simulink model "IMC_Ex1_simulink"  (R2018b)
settings: Solver=VariableStepAuto  StartTime=0.0  StopTime=4  RelTol=1e-3
values from neighbouring files (symbols this model uses):
  Kc = vars(5)    [Optimum.m]
  N = vars(4)    [CC.m]    (also in CHR.m; Optimum.m; PID_1.m = 10; PID_10.m = 10)
  Td = ((0.27-0.36*tau)/(1-0.87*tau)) * L    [CC.m]    (also in CHR.m = KK(typ, 6) * L; FOIPDT.m = T; IPDT.m = a(iC, 5) * L; Optimum.m = 0.144 * Tc)
  Ti = ((2.5-2*tau)/(1-0.39*tau)) * L    [CC.m]    (also in CHR.m = KK(typ, 5) * TT; FOIPDT.m = 2 * L * (1+a); IPDT.m = a(iC, 4) * L; Optimum.m = Tc * (1.751*kappa-0.612) / (3.776*kappa+1.388))
undefined symbols (not defined in the file or in its folder): b, c, N0, Tt, Tt0
settings Model: Creator=Erfan Etesami  LastModifiedBy=Erfan Etesami

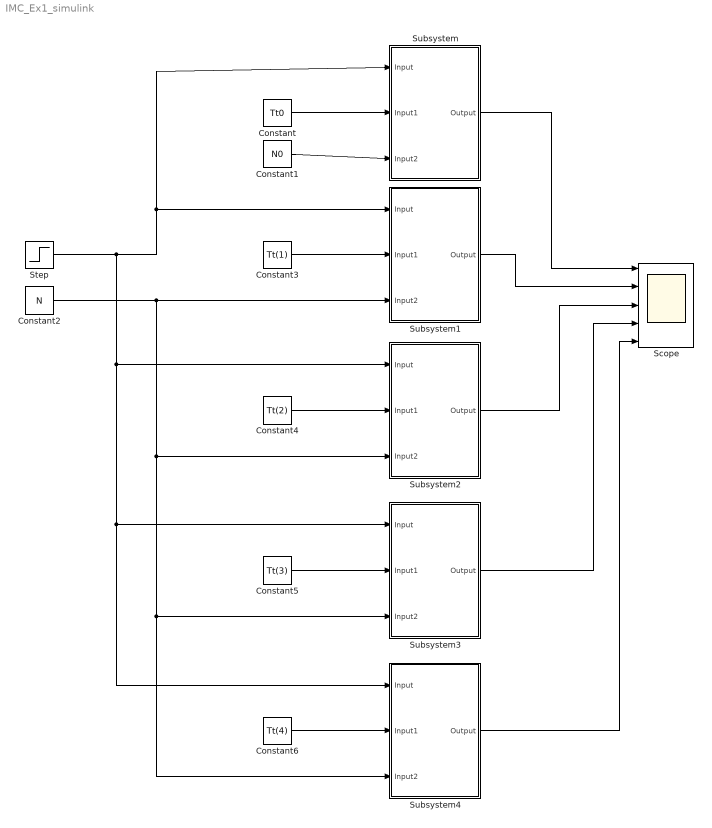
== system IMC_Ex1_simulink ==
  Constant : Constant  Value=Tt0
  Constant1 : Constant  Value=N0
  Constant2 : Constant  Value=N
  Constant3 : Constant  Value=Tt(1)
  Constant4 : Constant  Value=Tt(2)
  Constant5 : Constant  Value=Tt(3)
  Constant6 : Constant  Value=Tt(4)
  Scope : Scope  NumInputPorts=5
  Step : Step  Time=0  SampleTime=0
  Subsystem : Subsystem
  Subsystem1 : Subsystem
  Subsystem2 : Subsystem
  Subsystem3 : Subsystem
  Subsystem4 : Subsystem
  wires:
  Subsystem/1(Output) -> Scope/1
  Step/1 -> Subsystem/1(Input), Subsystem1/1(Input), Subsystem2/1(Input), Subsystem4/1(Input), Subsystem3/1(Input)
  Constant/1 -> Subsystem/2(Input1)
  Constant1/1 -> Subsystem/3(Input2)
  Constant2/1 -> Subsystem1/3(Input2), Subsystem2/3(Input2), Subsystem4/3(Input2), Subsystem3/3(Input2)
  Constant3/1 -> Subsystem1/2(Input1)
  Constant4/1 -> Subsystem2/2(Input1)
  Subsystem1/1(Output) -> Scope/2
  Subsystem2/1(Output) -> Scope/3
  Constant5/1 -> Subsystem3/2(Input1)
  Subsystem3/1(Output) -> Scope/4
  Constant6/1 -> Subsystem4/2(Input1)
  Subsystem4/1(Output) -> Scope/5

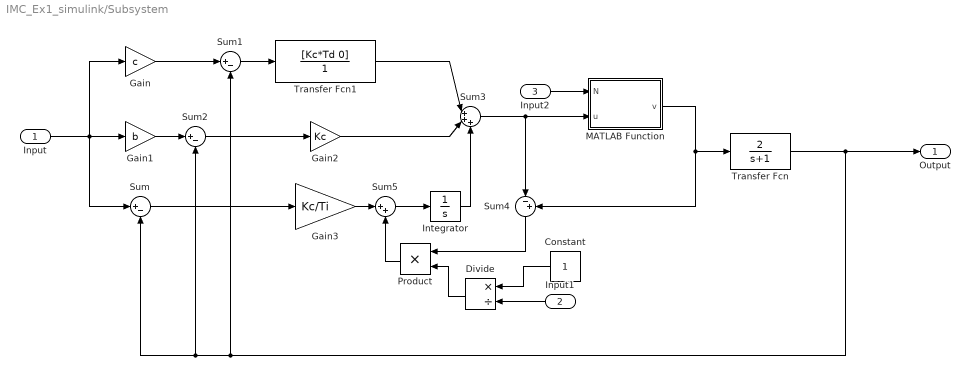
== system IMC_Ex1_simulink/Subsystem ==
  Input : Inport
  Input1 : Inport  Port=2
  Input2 : Inport  Port=3
  Constant : Constant
  Divide : Product  Inputs=*/
  Gain : Gain  Gain=c
  Gain1 : Gain  Gain=b
  Gain2 : Gain  Gain=Kc
  Gain3 : Gain  Gain=Kc/Ti
  Integrator : Integrator
  MATLAB Function : MATLAB Function  TreatAsAtomicUnit=on
  Product : Product
  Sum : Sum  Inputs=|+-
  Sum1 : Sum  Inputs=|+-
  Sum2 : Sum  Inputs=|+-
  Sum3 : Sum  Inputs=|+++
  Sum4 : Sum  Inputs=|-+
  Sum5 : Sum  Inputs=|++
  Transfer Fcn : TransferFcn  Numerator=[2]  Denominator=[1 1]
  Transfer Fcn1 : TransferFcn  Numerator=[Kc*Td 0]  Denominator=[1]
  Output : Outport
  wires:
  Product/1 -> Sum5/2
  Divide/1 -> Product/2
  Transfer Fcn/1 -> Output/1, Sum1/2, Sum2/2, Sum/2
  Input1/1 -> Divide/2
  MATLAB Function/1(v) -> Sum4/2, Transfer Fcn/1
  Input/1 -> Gain/1, Sum/1, Gain1/1
  Sum3/1 -> MATLAB Function/2(u), Sum4/1
  Transfer Fcn1/1 -> Sum3/1
  Gain/1 -> Sum1/1
  Constant/1 -> Divide/1
  Sum5/1 -> Integrator/1
  Sum4/1 -> Product/1
  Sum2/1 -> Gain2/1
  Gain3/1 -> Sum5/1
  Gain1/1 -> Sum2/1
  Integrator/1 -> Sum3/3
  Gain2/1 -> Sum3/2
  Sum/1 -> Gain3/1
  Sum1/1 -> Transfer Fcn1/1
  Input2/1 -> MATLAB Function/1(N)

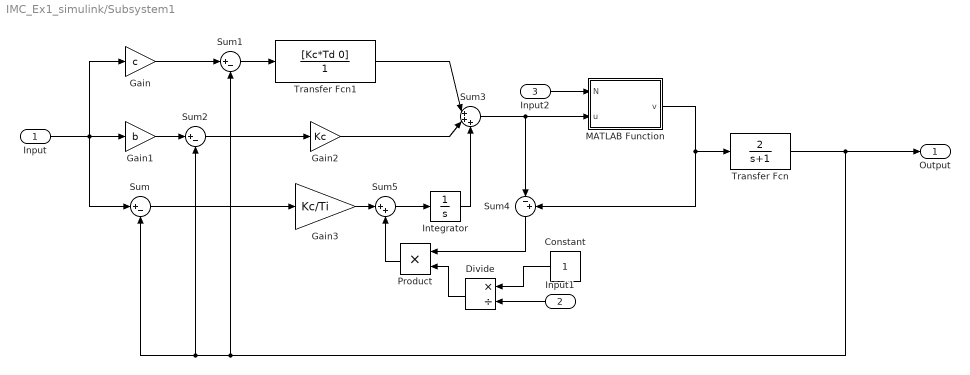
== system IMC_Ex1_simulink/Subsystem1 ==
  Input : Inport
  Input1 : Inport  Port=2
  Input2 : Inport  Port=3
  Constant : Constant
  Divide : Product  Inputs=*/
  Gain : Gain  Gain=c
  Gain1 : Gain  Gain=b
  Gain2 : Gain  Gain=Kc
  Gain3 : Gain  Gain=Kc/Ti
  Integrator : Integrator
  MATLAB Function : MATLAB Function  TreatAsAtomicUnit=on
  Product : Product
  Sum : Sum  Inputs=|+-
  Sum1 : Sum  Inputs=|+-
  Sum2 : Sum  Inputs=|+-
  Sum3 : Sum  Inputs=|+++
  Sum4 : Sum  Inputs=|-+
  Sum5 : Sum  Inputs=|++
  Transfer Fcn : TransferFcn  Numerator=[2]  Denominator=[1 1]
  Transfer Fcn1 : TransferFcn  Numerator=[Kc*Td 0]  Denominator=[1]
  Output : Outport
  wires:
  Input2/1 -> MATLAB Function/1(N)
  Sum1/1 -> Transfer Fcn1/1
  Sum/1 -> Gain3/1
  Gain2/1 -> Sum3/2
  Integrator/1 -> Sum3/3
  Gain1/1 -> Sum2/1
  Gain3/1 -> Sum5/1
  Sum2/1 -> Gain2/1
  Sum4/1 -> Product/1
  Sum5/1 -> Integrator/1
  Constant/1 -> Divide/1
  Gain/1 -> Sum1/1
  Transfer Fcn1/1 -> Sum3/1
  Sum3/1 -> Sum4/1, MATLAB Function/2(u)
  Input/1 -> Gain1/1, Sum/1, Gain/1
  MATLAB Function/1(v) -> Transfer Fcn/1, Sum4/2
  Input1/1 -> Divide/2
  Transfer Fcn/1 -> Sum/2, Sum2/2, Sum1/2, Output/1
  Divide/1 -> Product/2
  Product/1 -> Sum5/2

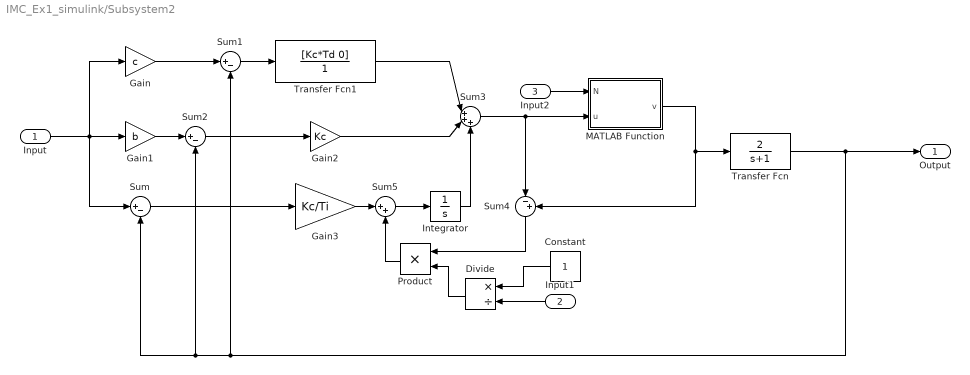
== system IMC_Ex1_simulink/Subsystem2 ==
  Input : Inport
  Input1 : Inport  Port=2
  Input2 : Inport  Port=3
  Constant : Constant
  Divide : Product  Inputs=*/
  Gain : Gain  Gain=c
  Gain1 : Gain  Gain=b
  Gain2 : Gain  Gain=Kc
  Gain3 : Gain  Gain=Kc/Ti
  Integrator : Integrator
  MATLAB Function : MATLAB Function  TreatAsAtomicUnit=on
  Product : Product
  Sum : Sum  Inputs=|+-
  Sum1 : Sum  Inputs=|+-
  Sum2 : Sum  Inputs=|+-
  Sum3 : Sum  Inputs=|+++
  Sum4 : Sum  Inputs=|-+
  Sum5 : Sum  Inputs=|++
  Transfer Fcn : TransferFcn  Numerator=[2]  Denominator=[1 1]
  Transfer Fcn1 : TransferFcn  Numerator=[Kc*Td 0]  Denominator=[1]
  Output : Outport
  wires:
  Product/1 -> Sum5/2
  Divide/1 -> Product/2
  Transfer Fcn/1 -> Output/1, Sum1/2, Sum2/2, Sum/2
  Input1/1 -> Divide/2
  MATLAB Function/1(v) -> Sum4/2, Transfer Fcn/1
  Input/1 -> Gain/1, Sum/1, Gain1/1
  Sum3/1 -> MATLAB Function/2(u), Sum4/1
  Transfer Fcn1/1 -> Sum3/1
  Gain/1 -> Sum1/1
  Constant/1 -> Divide/1
  Sum5/1 -> Integrator/1
  Sum4/1 -> Product/1
  Sum2/1 -> Gain2/1
  Gain3/1 -> Sum5/1
  Gain1/1 -> Sum2/1
  Integrator/1 -> Sum3/3
  Gain2/1 -> Sum3/2
  Sum/1 -> Gain3/1
  Sum1/1 -> Transfer Fcn1/1
  Input2/1 -> MATLAB Function/1(N)

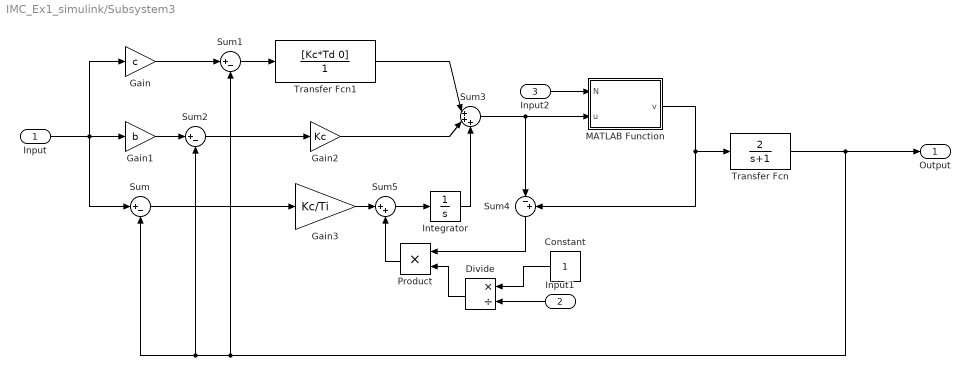
== system IMC_Ex1_simulink/Subsystem3 ==
  Input : Inport
  Input1 : Inport  Port=2
  Input2 : Inport  Port=3
  Constant : Constant
  Divide : Product  Inputs=*/
  Gain : Gain  Gain=c
  Gain1 : Gain  Gain=b
  Gain2 : Gain  Gain=Kc
  Gain3 : Gain  Gain=Kc/Ti
  Integrator : Integrator
  MATLAB Function : MATLAB Function  TreatAsAtomicUnit=on
  Product : Product
  Sum : Sum  Inputs=|+-
  Sum1 : Sum  Inputs=|+-
  Sum2 : Sum  Inputs=|+-
  Sum3 : Sum  Inputs=|+++
  Sum4 : Sum  Inputs=|-+
  Sum5 : Sum  Inputs=|++
  Transfer Fcn : TransferFcn  Numerator=[2]  Denominator=[1 1]
  Transfer Fcn1 : TransferFcn  Numerator=[Kc*Td 0]  Denominator=[1]
  Output : Outport
  wires:
  Input2/1 -> MATLAB Function/1(N)
  Sum1/1 -> Transfer Fcn1/1
  Sum/1 -> Gain3/1
  Gain2/1 -> Sum3/2
  Integrator/1 -> Sum3/3
  Gain1/1 -> Sum2/1
  Gain3/1 -> Sum5/1
  Sum2/1 -> Gain2/1
  Sum4/1 -> Product/1
  Sum5/1 -> Integrator/1
  Constant/1 -> Divide/1
  Gain/1 -> Sum1/1
  Transfer Fcn1/1 -> Sum3/1
  Sum3/1 -> Sum4/1, MATLAB Function/2(u)
  Input/1 -> Gain1/1, Sum/1, Gain/1
  MATLAB Function/1(v) -> Transfer Fcn/1, Sum4/2
  Input1/1 -> Divide/2
  Transfer Fcn/1 -> Sum/2, Sum2/2, Sum1/2, Output/1
  Divide/1 -> Product/2
  Product/1 -> Sum5/2

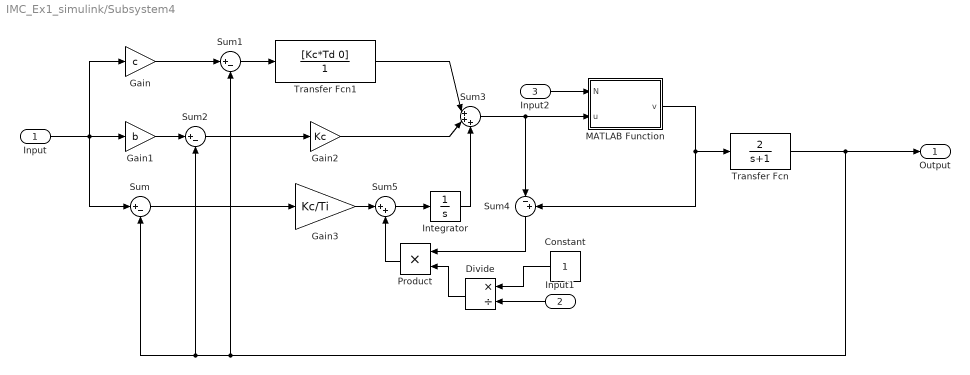
== system IMC_Ex1_simulink/Subsystem4 ==
  Input : Inport
  Input1 : Inport  Port=2
  Input2 : Inport  Port=3
  Constant : Constant
  Divide : Product  Inputs=*/
  Gain : Gain  Gain=c
  Gain1 : Gain  Gain=b
  Gain2 : Gain  Gain=Kc
  Gain3 : Gain  Gain=Kc/Ti
  Integrator : Integrator
  MATLAB Function : MATLAB Function  TreatAsAtomicUnit=on
  Product : Product
  Sum : Sum  Inputs=|+-
  Sum1 : Sum  Inputs=|+-
  Sum2 : Sum  Inputs=|+-
  Sum3 : Sum  Inputs=|+++
  Sum4 : Sum  Inputs=|-+
  Sum5 : Sum  Inputs=|++
  Transfer Fcn : TransferFcn  Numerator=[2]  Denominator=[1 1]
  Transfer Fcn1 : TransferFcn  Numerator=[Kc*Td 0]  Denominator=[1]
  Output : Outport
  wires:
  Product/1 -> Sum5/2
  Divide/1 -> Product/2
  Transfer Fcn/1 -> Output/1, Sum1/2, Sum2/2, Sum/2
  Input1/1 -> Divide/2
  MATLAB Function/1(v) -> Sum4/2, Transfer Fcn/1
  Input/1 -> Gain/1, Sum/1, Gain1/1
  Sum3/1 -> MATLAB Function/2(u), Sum4/1
  Transfer Fcn1/1 -> Sum3/1
  Gain/1 -> Sum1/1
  Constant/1 -> Divide/1
  Sum5/1 -> Integrator/1
  Sum4/1 -> Product/1
  Sum2/1 -> Gain2/1
  Gain3/1 -> Sum5/1
  Gain1/1 -> Sum2/1
  Integrator/1 -> Sum3/3
  Gain2/1 -> Sum3/2
  Sum/1 -> Gain3/1
  Sum1/1 -> Transfer Fcn1/1
  Input2/1 -> MATLAB Function/1(N)

== matlab function IMC_Ex1_simulink/Subsystem1/MATLAB Function ==
  data: N input; u input; v output
function v = fcn(N, u)

v = min(N, max(-N, u));

end

== matlab function IMC_Ex1_simulink/Subsystem/MATLAB Function ==
  data: N input; u input; v output
function v = fcn(N, u)

v = min(N, max(-N, u));

end

== matlab function IMC_Ex1_simulink/Subsystem2/MATLAB Function ==
  data: N input; u input; v output
function v = fcn(N, u)

v = min(N, max(-N, u));

end

== matlab function IMC_Ex1_simulink/Subsystem3/MATLAB Function ==
  data: N input; u input; v output
function v = fcn(N, u)

v = min(N, max(-N, u));

end

== matlab function IMC_Ex1_simulink/Subsystem4/MATLAB Function ==
  data: N input; u input; v output
function v = fcn(N, u)

v = min(N, max(-N, u));

end
